simulink model "sum"  (Simulink 6.6)
settings: Solver=FixedStepDiscrete  StartTime=0.0  StopTime=10.0  FixedStep=1  RelTol=1e-3
settings Model: Creator=ksmyth  LastModifiedBy=ksmyth

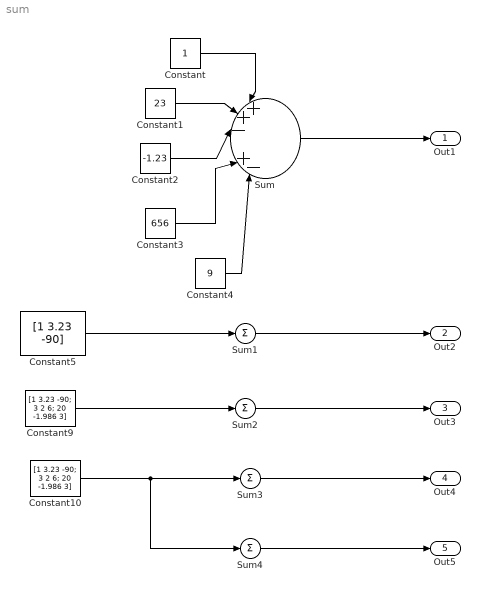
== system sum ==
  Constant : Constant
  Constant1 : Constant  Value=23
  Constant10 : Constant  Value=[1 3.23 -90; 3 2 6; 20 -1.986 3]
  Constant2 : Constant  Value=-1.23
  Constant3 : Constant  Value=656
  Constant4 : Constant  Value=9
  Constant5 : Constant  Value=[1 3.23 -90]
  Constant9 : Constant  Value=[1 3.23 -90; 3 2 6; 20 -1.986 3]
  Sum : Sum  Inputs=|++-|+-|
  Sum1 : Sum  Inputs=1
  Sum2 : Sum  Inputs=1
  Sum3 : Sum  Inputs=1  CollapseMode=Specified dimension
  Sum4 : Sum  Inputs=1  CollapseMode=Specified dimension  CollapseDim=2
  Out1 : Outport
  Out2 : Outport  Port=2
  Out3 : Outport  Port=3
  Out4 : Outport  Port=4
  Out5 : Outport  Port=5
  wires:
  Constant/1 -> Sum/1
  Constant1/1 -> Sum/2
  Constant2/1 -> Sum/3
  Constant3/1 -> Sum/4
  Constant4/1 -> Sum/5
  Sum/1 -> Out1/1
  Constant5/1 -> Sum1/1
  Sum1/1 -> Out2/1
  Constant9/1 -> Sum2/1
  Sum2/1 -> Out3/1
  Constant10/1 -> Sum3/1, Sum4/1
  Sum3/1 -> Out4/1
  Sum4/1 -> Out5/1
